simulink model "k1visitmyp"  (Simulink 8.8)
settings: Solver=ode45  StartTime=0.0  StopTime=10.0  RelTol=1e-3  EnableMultiTasking=on
libraries: cdsIPCx x7, cdsCDI64 x6, cdsCDO64 x6, dac x3, PAYLOAD_MASTER x3, cdsAdcx0 x1, cdsAdcx1 x1, cdsAdcx2 x1, BIO_CD_ENCODE_MASTER x1, BIO_CD_DECODE_MASTER x1, cdsParameters x1
settings Model: SuppressorTable=22 serialization::archive 11 0 3 0 0 0 11 0  Creator=controls  LastModifiedBy=controls
settings DataIOCC: SignalLoggingSaveFormat=Dataset
settings DebuggingCC: UnderspecifiedInitializationDetection=Simplified  MergeDetectMultiDrivingBlocksExec=error  FcnCallInpInsideContextMsg=error  AllowSymbolicDim=off  StateNameClashWarn=none
settings GRTTargetCC: CombineOutputUpdateFcns=on  GRTInterface=off

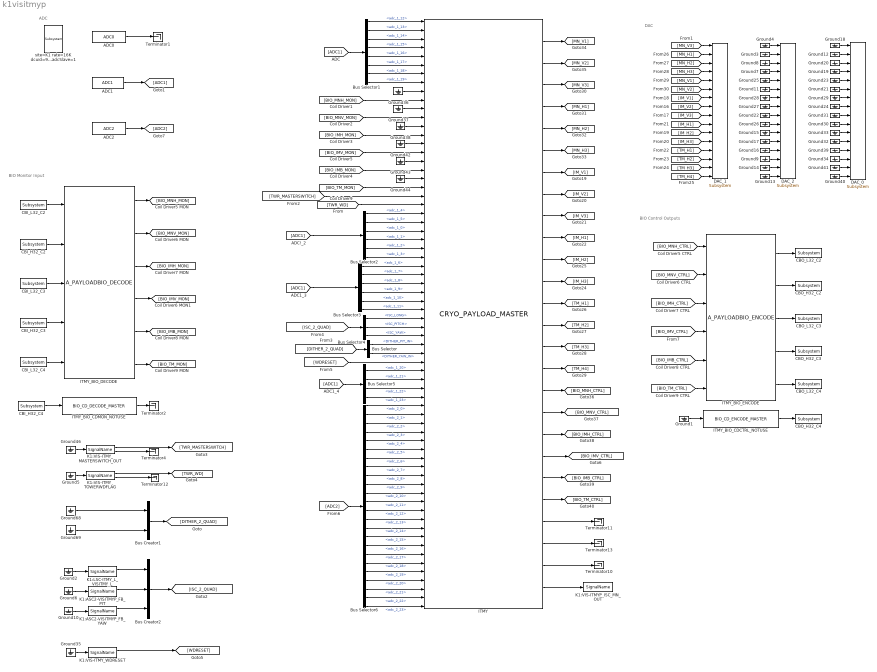
== system k1visitmyp ==
  note: BIO Monitor Input
  note: BIO Control Outputs
  note: DAC
  note: ADC
  ADC0 : cdsAdcx0/ADC0  Tag=cdsAdc  Description=|
      | type-GSC_16AI64SSA
      | card_num=0
      settings: AttributesFormatString=%<Description>\n%<Tag>
  ADC1 : cdsAdcx1/ADC1  Tag=cdsAdc  Description=|
      | type-GSC_16AI64SSA
      | card_num=1
      settings: AttributesFormatString=%<Description>\n%<Tag>
  ADC2 : cdsAdcx2/ADC2  Tag=cdsAdc  Description=|
      | type-GSC_16AI64SSA
      | card_num=2
      settings: AttributesFormatString=%<Description>\n%<Tag>
  Bus Creator1 : BusCreator  Inputs='DITHER_PIT_IN','DITHER_YAW_IN'
  Bus Creator2 : BusCreator  Inputs='ISC_LONG','ISC_PITCH','ISC_YAW'
  Bus Selector : BusSelector  OutputSignals=DITHER_PIT_IN,DITHER_YAW_IN
  Bus Selector1 : BusSelector  OutputSignals=adc_1_12,adc_1_13,adc_1_14,adc_1_15,adc_1_16,adc_1_17,adc_1_18,adc_1_19
  Bus Selector2 : BusSelector  OutputSignals=adc_1_4,adc_1_5,adc_1_0,adc_1_1,adc_1_2,adc_1_3
  Bus Selector3 : BusSelector  OutputSignals=adc_1_6,adc_1_7,adc_1_8,adc_1_9,adc_1_10,adc_1_11
  Bus Selector4 : BusSelector  OutputSignals=ISC_LONG,ISC_PITCH,ISC_YAW
  Bus Selector5 : BusSelector  OutputSignals=adc_1_20,adc_1_21,adc_1_22,adc_1_23
  Bus Selector6 : BusSelector  OutputSignals=adc_2_0,adc_2_1,adc_2_2,adc_2_3,adc_2_4,adc_2_5,adc_2_6,adc_2_7,adc_2_8,adc_2_9,adc_2_10,adc_2_11,adc_2_12,adc_2_13,adc_2_14,adc_2_15,adc_2_16,adc_2_17,adc_2_18,adc_2_19,adc_2_20,adc_2_21,adc_2_22,adc_2_23
  CBI_H32_C2 : cdsCDI64/Subsystem  Tag=cdsCDI64  Description=card_num=5
      settings: AttributesFormatString=%<Tag>\n%<Description>
  CBI_H32_C3 : cdsCDI64/Subsystem  Tag=cdsCDI64  Description=card_num=7
      settings: AttributesFormatString=%<Tag>\n%<Description>
  CBI_H32_C4 : cdsCDI64/Subsystem  Tag=cdsCDI64  Description=card_num=9
      settings: AttributesFormatString=%<Tag>\n%<Description>
  CBI_L32_C2 : cdsCDI64/Subsystem  Tag=cdsCDI64  Description=card_num=4
      settings: AttributesFormatString=%<Tag>\n%<Description>
  CBI_L32_C3 : cdsCDI64/Subsystem  Tag=cdsCDI64  Description=card_num=6
      settings: AttributesFormatString=%<Tag>\n%<Description>
  CBI_L32_C4 : cdsCDI64/Subsystem  Tag=cdsCDI64  Description=card_num=8
      settings: AttributesFormatString=%<Tag>\n%<Description>
  CBO_H32_C2 : cdsCDO64/Subsystem  Tag=cdsCDO64  Description=card_num=5
      settings: AttributesFormatString=%<Tag>\n%<Description>
  CBO_H32_C3 : cdsCDO64/Subsystem  Tag=cdsCDO64  Description=card_num=7
      settings: AttributesFormatString=%<Tag>\n%<Description>
  CBO_H32_C4 : cdsCDO64/Subsystem  Tag=cdsCDO64  Description=card_num=9
      settings: AttributesFormatString=%<Tag>\n%<Description>
  CBO_L32_C2 : cdsCDO64/Subsystem  Tag=cdsCDO64  Description=card_num=4
      settings: AttributesFormatString=%<Tag>\n%<Description>
  CBO_L32_C3 : cdsCDO64/Subsystem  Tag=cdsCDO64  Description=card_num=6
      settings: AttributesFormatString=%<Tag>\n%<Description>
  CBO_L32_C4 : cdsCDO64/Subsystem  Tag=cdsCDO64  Description=card_num=8
      settings: AttributesFormatString=%<Tag>\n%<Description>
  DAC_0 : dac/Subsystem  Description=|
      | type=GSC_16AO16,
      | card_num=0
      settings: AttributesFormatString=%<Description>
  DAC_1 : dac/Subsystem  Description=|
      | type=GSC_16AO16,
      | card_num=1
      settings: AttributesFormatString=%<Description>
  DAC_2 : dac/Subsystem  Description=|
      | type=GSC_16AO16,
      | card_num=2
      settings: AttributesFormatString=%<Description>
  Ground{1..44,46,68..69} (47 alike) : Ground
  ITMY : PAYLOAD_MASTER/CRYO_PAYLOAD_MASTER
  ITMY_BIO_CDCTRL_NOTUSE : BIO_CD_ENCODE_MASTER/BIO_CD_ENCODE_MASTER
  ITMY_BIO_CDMON_NOTUSE : BIO_CD_DECODE_MASTER/BIO_CD_DECODE_MASTER
  ITMY_BIO_DECODE : PAYLOAD_MASTER/A_PAYLOADBIO_DECODE
  ITMY_BIO_ENCODE : PAYLOAD_MASTER/A_PAYLOADBIO_ENCODE
  K1:ASC2-VISITMYP_FB_PIT : cdsIPCx/SignalName  Tag=cdsIPCx_RFM  Description=card=1
      settings: AttributesFormatString=%<Description>\n%<Tag>
  K1:ASC2-VISITMYP_FB_YAW : cdsIPCx/SignalName  Tag=cdsIPCx_RFM  Description=card=1
      settings: AttributesFormatString=%<Description>\n%<Tag>
  K1:LSC-ITMY_L_VISITMY_L : cdsIPCx/SignalName  Tag=cdsIPCx_RFM  Description=card=1
      settings: AttributesFormatString=%<Description>\n%<Tag>
  K1:VIS-ITMYP_ISC_MN_OUT : cdsIPCx/SignalName  Tag=cdsIPCx_SHMEM  Description=Inter-Process Communication via Shared memory.
      settings: AttributesFormatString=%<Tag>
  K1:VIS-ITMY_MASTERSWITCH_OUT : cdsIPCx/SignalName  Tag=cdsIPCx_SHMEM  Description=Inter-Process Communication via Shared memory.
      settings: AttributesFormatString=%<Tag>
  K1:VIS-ITMY_TOWERWDFLAG : cdsIPCx/SignalName  Tag=cdsIPCx_SHMEM  Description=Inter-Process Communication via Shared memory.
      settings: AttributesFormatString=%<Tag>
  K1:VIS-ITMY_WDRESET : cdsIPCx/SignalName  Tag=cdsIPCx_SHMEM  Description=Inter-Process Communication via Shared memory.
      settings: AttributesFormatString=%<Tag>
  Terminator{1..2,4,10..13} (7 alike) : Terminator
  site=K1 rate=16K dcuid=98 host=k1iy1 specific_cpu=3 adcSlave=1 : cdsParameters/Subsystem  Tag=cdsParameters  Description=|
      | Purpose:                                                                                                                                                                                                                                
      | Provide system parameters to the FE code generator to properly configure the generated EPICS names, rep rate of the FE controller, and the Data Acquisition node ID for proper storage of data from this FE controller.                 
      |                                                                                                                                                                                                                                         
      | Useage:                                                                                                                                                                                                                                 
      | The part NAME field is used to identify the FE parameters. It must be of the form:                                                                                                                                                      
      | site=                                                                                                                                                                                                                                   
      | rate=                                                                                                                                                                                                                                   
      | dcuid=                                                                                                                                                                                                                                  
      |                                                                                                                                                                                                                                         
      | Where:                                                                                                                                                                                                                                  
      | site= argument may be H1, H2, L1, M1, G1, either as a single argument or multiple, for example site=H1,H2. These are the only names allowed. These will become the first two characters of all EPICS and signal names (for example G1:).
      |                                                                                                                                                                                                                                         
      | rate= may be 2K, 16K, 32K, or 64K                                                                                                                                                                                                       
      |                                                                                                                                                                                                                                         
      | dcuid= is site specific ie it must be unique at each site.
      settings: AttributesFormatString=%<Tag>
  wires:
  ADC1/1 -> [ADC1]
  [MN_V3] -> DAC_1/1
  [MN_H1] -> DAC_1/2
  [MN_H2] -> DAC_1/3
  [MN_H3] -> DAC_1/4
  [MN_V1] -> DAC_1/5
  [MN_V2] -> DAC_1/6
  [IM_V1] -> DAC_1/7
  [IM_V2] -> DAC_1/8
  [IM_V3] -> DAC_1/9
  [IM_H1] -> DAC_1/10
  [TM_H1] -> DAC_1/13
  [TM_H4] -> DAC_1/16
  [TM_H3] -> DAC_1/15
  [TM_H2] -> DAC_1/14
  [IM_H2] -> DAC_1/11
  [IM_H3] -> DAC_1/12
  [BIO_MNH_CTRL] -> ITMY_BIO_ENCODE/1
  ITMY_BIO_ENCODE/1 -> CBO_L32_C2/1
  [BIO_MNV_CTRL] -> ITMY_BIO_ENCODE/2
  ITMY_BIO_ENCODE/2 -> CBO_H32_C2/1
  [BIO_IMH_CTRL] -> ITMY_BIO_ENCODE/3
  ITMY_BIO_ENCODE/3 -> CBO_L32_C3/1
  [BIO_IMB_CTRL] -> ITMY_BIO_ENCODE/5
  ITMY_BIO_ENCODE/4 -> CBO_H32_C3/1
  [BIO_TM_CTRL] -> ITMY_BIO_ENCODE/6
  ITMY_BIO_ENCODE/5 -> CBO_L32_C4/1
  Ground1/1 -> ITMY_BIO_CDCTRL_NOTUSE/1
  ITMY_BIO_CDCTRL_NOTUSE/1 -> CBO_H32_C4/1
  CBI_L32_C2/1 -> ITMY_BIO_DECODE/1
  ITMY_BIO_DECODE/1 -> [BIO_MNH_MON]
  CBI_H32_C2/1 -> ITMY_BIO_DECODE/2
  ITMY_BIO_DECODE/2 -> [BIO_MNV_MON]
  CBI_L32_C3/1 -> ITMY_BIO_DECODE/3
  ITMY_BIO_DECODE/3 -> [BIO_IMH_MON]
  ITMY_BIO_DECODE/5 -> [BIO_IMB_MON]
  CBI_L32_C4/1 -> ITMY_BIO_DECODE/5
  ITMY_BIO_DECODE/6 -> [BIO_TM_MON]
  CBI_H32_C4/1 -> ITMY_BIO_CDMON_NOTUSE/1
  ITMY_BIO_CDMON_NOTUSE/1 -> Terminator2/1
  Ground4/1 -> DAC_2/1
  Ground3/1 -> DAC_2/2
  Ground8/1 -> DAC_2/3
  Ground7/1 -> DAC_2/4
  Ground25/1 -> DAC_2/5
  Ground11/1 -> DAC_2/6
  Ground28/1 -> DAC_2/7
  Ground27/1 -> DAC_2/8
  Ground22/1 -> DAC_2/9
  Ground26/1 -> DAC_2/10
  Ground15/1 -> DAC_2/11
  Ground17/1 -> DAC_2/12
  Ground16/1 -> DAC_2/13
  Ground9/1 -> DAC_2/14
  Ground14/1 -> DAC_2/15
  Ground13/1 -> DAC_2/16
  CBI_H32_C3/1 -> ITMY_BIO_DECODE/4
  [ADC1] -> Bus Selector1/1
  K1:VIS-ITMY_TOWERWDFLAG/2 -> Terminator12/1
  Ground5/1 -> K1:VIS-ITMY_TOWERWDFLAG/1
  ADC0/1 -> Terminator1/1
  Ground18/1 -> DAC_0/1
  Ground12/1 -> DAC_0/2
  Ground19/1 -> DAC_0/4
  Ground20/1 -> DAC_0/3
  Ground29/1 -> DAC_0/7
  Ground23/1 -> DAC_0/5
  Ground21/1 -> DAC_0/6
  Ground24/1 -> DAC_0/8
  Ground31/1 -> DAC_0/9
  Ground30/1 -> DAC_0/10
  Ground33/1 -> DAC_0/11
  Ground32/1 -> DAC_0/12
  Ground39/1 -> DAC_0/13
  Ground34/1 -> DAC_0/14
  Ground41/1 -> DAC_0/15
  Ground40/1 -> DAC_0/16
  Ground46/1 -> K1:VIS-ITMY_MASTERSWITCH_OUT/1
  K1:VIS-ITMY_MASTERSWITCH_OUT/2 -> Terminator4/1
  Ground36/1 -> ITMY/9
  [BIO_MNH_MON] -> ITMY/10
  Ground37/1 -> ITMY/11
  [BIO_MNV_MON] -> ITMY/12
  Ground38/1 -> ITMY/13
  [BIO_IMH_MON] -> ITMY/14
  Ground43/1 -> ITMY/17
  [BIO_IMB_MON] -> ITMY/18
  Ground44/1 -> ITMY/19
  [BIO_TM_MON] -> ITMY/20
  ITMY/2 -> [MN_V2]
  ITMY/1 -> [MN_V1]
  ITMY/3 -> [MN_V3]
  ITMY/4 -> [MN_H1]
  ITMY/5 -> [MN_H2]
  ITMY/6 -> [MN_H3]
  ITMY/7 -> [IM_V1]
  ITMY/8 -> [IM_V2]
  ITMY/9 -> [IM_V3]
  ITMY/10 -> [IM_H1]
  ITMY/11 -> [IM_H2]
  ITMY/12 -> [IM_H3]
  ITMY/13 -> [TM_H1]
  ITMY/14 -> [TM_H2]
  ITMY/15 -> [TM_H3]
  ITMY/19 -> [BIO_IMH_CTRL]
  ITMY/18 -> [BIO_MNV_CTRL]
  ITMY/17 -> [BIO_MNH_CTRL]
  ITMY/16 -> [TM_H4]
  ITMY/21 -> [BIO_IMB_CTRL]
  ITMY/22 -> [BIO_TM_CTRL]
  Bus Selector1/1 -> ITMY/1  "<adc_1_12>"
  Bus Selector1/2 -> ITMY/2  "<adc_1_13>"
  Bus Selector1/3 -> ITMY/3  "<adc_1_14>"
  Bus Selector1/4 -> ITMY/4  "<adc_1_15>"
  Bus Selector1/5 -> ITMY/5  "<adc_1_16>"
  Bus Selector1/6 -> ITMY/6  "<adc_1_17>"
  Bus Selector1/7 -> ITMY/7  "<adc_1_18>"
  Bus Selector1/8 -> ITMY/8  "<adc_1_19>"
  K1:VIS-ITMY_TOWERWDFLAG/1 -> [TWR_WD]
  K1:VIS-ITMY_MASTERSWITCH_OUT/1 -> [TWR_MASTERSWITCH]
  [TWR_MASTERSWITCH] -> ITMY/21
  [TWR_WD] -> ITMY/22
  [ADC1] -> Bus Selector2/1
  Bus Selector2/1 -> ITMY/23  "<adc_1_4>"
  Bus Selector2/2 -> ITMY/24  "<adc_1_5>"
  Bus Selector2/3 -> ITMY/25  "<adc_1_0>"
  Bus Selector2/4 -> ITMY/26  "<adc_1_1>"
  Bus Selector2/5 -> ITMY/27  "<adc_1_2>"
  Bus Selector2/6 -> ITMY/28  "<adc_1_3>"
  [ADC1] -> Bus Selector3/1
  Bus Selector3/1 -> ITMY/29  "<adc_1_6>"
  Bus Selector3/2 -> ITMY/30  "<adc_1_7>"
  Bus Selector3/3 -> ITMY/31  "<adc_1_8>"
  Bus Selector3/4 -> ITMY/32  "<adc_1_9>"
  Bus Selector3/5 -> ITMY/33  "<adc_1_10>"
  Bus Selector3/6 -> ITMY/34  "<adc_1_11>"
  [DITHER_2_QUAD] -> Bus Selector/1
  [ISC_2_QUAD] -> Bus Selector4/1
  Bus Selector4/1 -> ITMY/35  "<ISC_LONG>"
  Bus Selector4/2 -> ITMY/36  "<ISC_PITCH>"
  Bus Selector4/3 -> ITMY/37  "<ISC_YAW>"
  [WDRESET] -> ITMY/40
  Bus Selector/1 -> ITMY/38  "<DITHER_PIT_IN>"
  Bus Selector/2 -> ITMY/39  "<DITHER_YAW_IN>"
  [ADC1] -> Bus Selector5/1
  Bus Selector5/1 -> ITMY/41  "<adc_1_20>"
  Bus Selector5/2 -> ITMY/42  "<adc_1_21>"
  Bus Selector5/3 -> ITMY/43  "<adc_1_22>"
  Bus Selector5/4 -> ITMY/44  "<adc_1_23>"
  [ADC2] -> Bus Selector6/1
  Bus Selector6/1 -> ITMY/45  "<adc_2_0>"
  Bus Selector6/2 -> ITMY/46  "<adc_2_1>"
  Bus Selector6/3 -> ITMY/47  "<adc_2_2>"
  Bus Selector6/4 -> ITMY/48  "<adc_2_3>"
  Bus Selector6/5 -> ITMY/49  "<adc_2_4>"
  Bus Selector6/6 -> ITMY/50  "<adc_2_5>"
  Bus Selector6/7 -> ITMY/51  "<adc_2_6>"
  Bus Selector6/8 -> ITMY/52  "<adc_2_7>"
  Bus Selector6/9 -> ITMY/53  "<adc_2_8>"
  Bus Selector6/10 -> ITMY/54  "<adc_2_9>"
  Bus Selector6/11 -> ITMY/55  "<adc_2_10>"
  Bus Selector6/12 -> ITMY/56  "<adc_2_11>"
  Bus Selector6/13 -> ITMY/57  "<adc_2_12>"
  Bus Selector6/14 -> ITMY/58  "<adc_2_13>"
  Bus Selector6/15 -> ITMY/59  "<adc_2_14>"
  Bus Selector6/16 -> ITMY/60  "<adc_2_15>"
  Bus Selector6/17 -> ITMY/61  "<adc_2_16>"
  Bus Selector6/18 -> ITMY/62  "<adc_2_17>"
  Bus Selector6/19 -> ITMY/63  "<adc_2_18>"
  Bus Selector6/20 -> ITMY/64  "<adc_2_19>"
  Bus Selector6/21 -> ITMY/65  "<adc_2_20>"
  Bus Selector6/22 -> ITMY/66  "<adc_2_21>"
  Bus Selector6/23 -> ITMY/67  "<adc_2_22>"
  Bus Selector6/24 -> ITMY/68  "<adc_2_23>"
  Ground6/1 -> K1:ASC2-VISITMYP_FB_PIT/1
  Ground10/1 -> K1:ASC2-VISITMYP_FB_YAW/1
  Ground2/1 -> K1:LSC-ITMY_L_VISITMY_L/1
  Bus Creator1/1 -> [DITHER_2_QUAD]
  Bus Creator2/1 -> [ISC_2_QUAD]
  K1:LSC-ITMY_L_VISITMY_L/1 -> Bus Creator2/1
  K1:ASC2-VISITMYP_FB_PIT/1 -> Bus Creator2/2
  K1:ASC2-VISITMYP_FB_YAW/1 -> Bus Creator2/3
  Ground68/1 -> Bus Creator1/1
  Ground69/1 -> Bus Creator1/2
  Ground35/1 -> K1:VIS-ITMY_WDRESET/1
  K1:VIS-ITMY_WDRESET/1 -> [WDRESET]
  ITMY/23 -> Terminator11/1
  ITMY/24 -> Terminator13/1
  ITMY/26 -> K1:VIS-ITMYP_ISC_MN_OUT/1
  ITMY/25 -> Terminator10/1
  ITMY/20 -> [BIO_IMV_CTRL]
  [BIO_IMV_CTRL] -> ITMY_BIO_ENCODE/4
  Ground42/1 -> ITMY/15
  [BIO_IMV_MON] -> ITMY/16
  ITMY_BIO_DECODE/4 -> [BIO_IMV_MON]
  ADC2/1 -> [ADC2]
